simulink model "color_palette_v3"  (Simulink 7.6)
settings: Solver=FixedStepDiscrete  StartTime=0.0  StopTime=0  FixedStep=1/30  RelTol=1e-3
values from neighbouring files (symbols this model uses):
  Iter_Segment_Thresh = 60    [VisionConstants.m]
  Scale_Forward_B = 1    [VisionConstants.m]
  Scale_Forward_G = 1    [VisionConstants.m]
  Scale_Forward_H = .8    (= 0.8)    [VisionConstants.m]
  Scale_Forward_R = 1    [VisionConstants.m]
  Scale_Forward_S = 1    [VisionConstants.m]
  Scale_Forward_V = 2    [VisionConstants.m]
undefined symbols (not defined in the file or in its folder): a_range, b_range, jet, Rec, SDTV
libraries: vipconversions x5, vipgeotforms x3, vipsnks x2, vipsrcs x1
settings Model: Creator=auvt  LastModifiedBy=auvt
settings RTWCC: TargetLang=C++

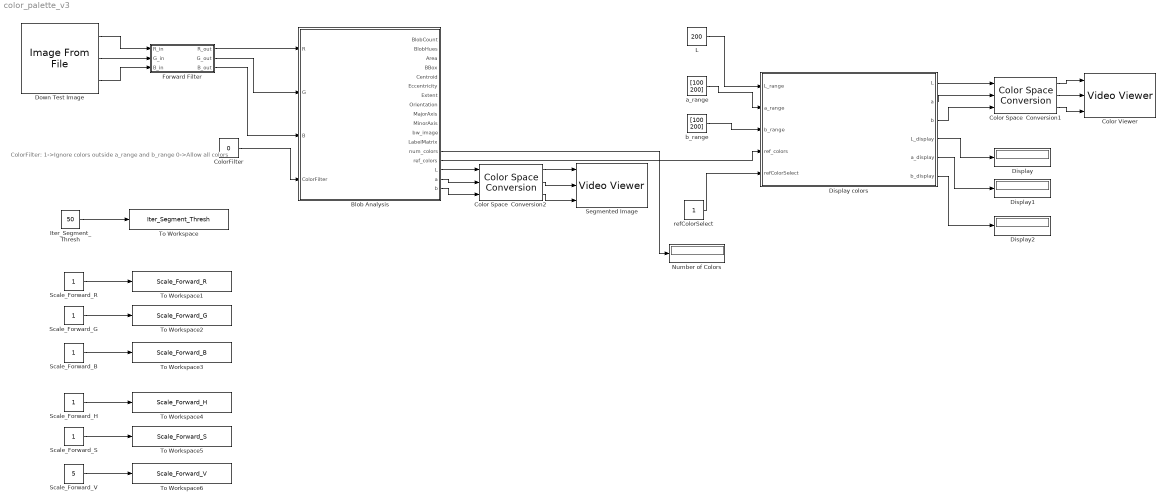
== system color_palette_v3 ==
  note: ColorFilter:
      | 1->Ignore colors outside a_range and b_range
      | 0->Allow all colors
  Blob Analysis : Subsystem
  Color Space  Conversion1 : vipconversions/Color Space  Conversion  conversion=Obsolete  conversionActive=L*a*b* to sR'G'B'  wp_str=D50  rec=Rec. 601 (SDTV)  sys=1125/60/2:1  imagePorts=Separate color signals
  Color Space  Conversion2 : vipconversions/Color Space  Conversion  conversion=Obsolete  conversionActive=L*a*b* to sR'G'B'  wp_str=D50  rec=Rec. 601 (SDTV)  sys=1125/60/2:1  imagePorts=Separate color signals
  Color Viewer : vipsnks/Video Viewer  DialogControllerArgs=DataTag4  inputType=Obsolete7b  imagePorts=Separate color signals  useColorMap=off  colormapValue=jet(256)  specRange=off  minInputVal=0  maxInputVal=255  FigPos=[1526 467 410 300]  AxisZoom=on  trueSizedOnce=off  OpenAtMdlStart=on
  ColorFilter : Constant  Value=0  SampleTime=-1
  Display : Display
  Display colors : Stateflow chart  TreatAsAtomicUnit=on  SystemSampleTime=[1/30 0]
  Display1 : Display
  Display2 : Display
  Down Test Image : vipsrcs/Image From File  Tag=vipblks_nd  DialogController=vipDDGCreate  DialogControllerArgs=DataTag5  SystemSampleTime=-1  FileName=/home/auvt/auvc/src/vision/Test_Images/gate10.bmp  imagePorts=Separate color signals  Ts=-1  ImageDataType=double  Signed=on  WordLength=16  sdImageDataType=uint(8)  FractionLengthMode=User-defined  FractionLength=15  OutPortLabels=R|G|B
  Forward Filter : Subsystem
  Iter_Segment_Thresh : Constant  Value=50  SampleTime=-1
  L : Constant  Value=200  SampleTime=-1
  Number of Colors : Display
  Scale_Forward_B : Constant  SampleTime=-1
  Scale_Forward_G : Constant  SampleTime=-1
  Scale_Forward_H : Constant  SampleTime=-1
  Scale_Forward_R : Constant  SampleTime=-1
  Scale_Forward_S : Constant  SampleTime=-1
  Scale_Forward_V : Constant  Value=5  SampleTime=-1
  Segmented Image : vipsnks/Video Viewer  DialogControllerArgs=DataTag7  inputType=Obsolete7b  imagePorts=Separate color signals  useColorMap=off  colormapValue=jet(256)  specRange=off  minInputVal=0  maxInputVal=255  FigPos=[1521 919 410 300]  AxisZoom=on  trueSizedOnce=off  OpenAtMdlStart=on
  To Workspace : ToWorkspace  VariableName=Iter_Segment_Thresh  SampleTime=-1  SaveFormat=Array
  To Workspace1 : ToWorkspace  VariableName=Scale_Forward_R  SampleTime=-1  SaveFormat=Array
  To Workspace2 : ToWorkspace  VariableName=Scale_Forward_G  SampleTime=-1  SaveFormat=Array
  To Workspace3 : ToWorkspace  VariableName=Scale_Forward_B  SampleTime=-1  SaveFormat=Array
  To Workspace4 : ToWorkspace  VariableName=Scale_Forward_H  SampleTime=-1  SaveFormat=Array
  To Workspace5 : ToWorkspace  VariableName=Scale_Forward_S  SampleTime=-1  SaveFormat=Array
  To Workspace6 : ToWorkspace  VariableName=Scale_Forward_V  SampleTime=-1  SaveFormat=Array
  a_range : Constant  Value=[100 200]  SampleTime=-1
  b_range : Constant  Value=[100 200]  SampleTime=-1
  refColorSelect : Constant  SampleTime=-1
  wires:
  Display colors/1(L) -> Color Space  Conversion1/1
  Display colors/2(a) -> Color Space  Conversion1/2
  Display colors/3(b) -> Color Space  Conversion1/3
  refColorSelect/1 -> Display colors/5(refColorSelect)
  ColorFilter/1 -> Blob Analysis/4(ColorFilter)
  Blob Analysis/14(ref_colors) -> Display colors/4(ref_colors)
  L/1 -> Display colors/1(L_range)
  a_range/1 -> Display colors/2(a_range)
  b_range/1 -> Display colors/3(b_range)
  Display colors/4(L_display) -> Display/1
  Display colors/5(a_display) -> Display1/1
  Display colors/6(b_display) -> Display2/1
  Blob Analysis/13(num_colors) -> Number of Colors/1
  Blob Analysis/15(L) -> Color Space  Conversion2/1
  Blob Analysis/16(a) -> Color Space  Conversion2/2
  Blob Analysis/17(b) -> Color Space  Conversion2/3
  Color Space  Conversion2/1 -> Segmented Image/1
  Color Space  Conversion2/2 -> Segmented Image/2
  Color Space  Conversion2/3 -> Segmented Image/3
  Iter_Segment_Thresh/1 -> To Workspace/1
  Forward Filter/1(R_out) -> Blob Analysis/1(R)
  Forward Filter/2(G_out) -> Blob Analysis/2(G)
  Forward Filter/3(B_out) -> Blob Analysis/3(B)
  Down Test Image/1 -> Forward Filter/1(R_in)
  Down Test Image/2 -> Forward Filter/2(G_in)
  Down Test Image/3 -> Forward Filter/3(B_in)
  Scale_Forward_R/1 -> To Workspace1/1
  Scale_Forward_G/1 -> To Workspace2/1
  Scale_Forward_B/1 -> To Workspace3/1
  Scale_Forward_H/1 -> To Workspace4/1
  Scale_Forward_S/1 -> To Workspace5/1
  Scale_Forward_V/1 -> To Workspace6/1
  Color Space  Conversion1/1 -> Color Viewer/1
  Color Space  Conversion1/2 -> Color Viewer/2
  Color Space  Conversion1/3 -> Color Viewer/3

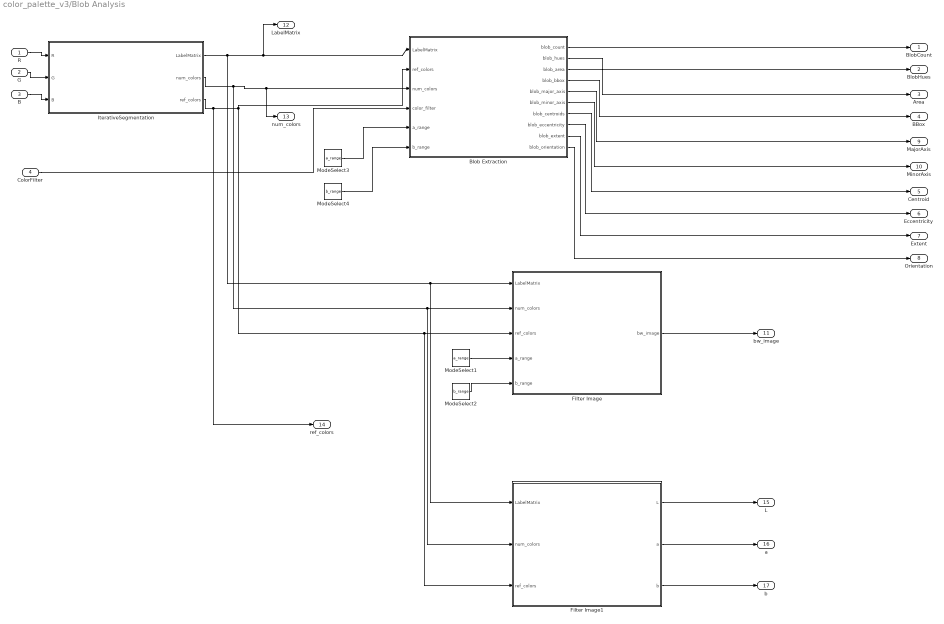
== system color_palette_v3/Blob Analysis ==
  R : Inport
  G : Inport  Port=2
  B : Inport  Port=3
  ColorFilter : Inport  Port=4
  Blob Extraction : Stateflow chart  TreatAsAtomicUnit=on
  Filter Image : Stateflow chart  TreatAsAtomicUnit=on
  Filter Image1 : Stateflow chart  TreatAsAtomicUnit=on
  IterativeSegmentation : Subsystem
      settings: UndoDeleteFcn=Stateflow.SLINSF.SimulinkMan.restorePreDeleteFcn  PreDeleteFcn=Stateflow.SLINSF.SimulinkMan.removePreDeleteFcn
  ModeSelect1 : Constant  Value=a_range  SampleTime=-1
  ModeSelect2 : Constant  Value=b_range  SampleTime=-1
  ModeSelect3 : Constant  Value=a_range  SampleTime=-1
  ModeSelect4 : Constant  Value=b_range  SampleTime=-1
  BlobCount : Outport
  BlobHues : Outport  Port=2
  Area : Outport  Port=3
  BBox : Outport  Port=4
  Centroid : Outport  Port=5
  Eccentricity : Outport  Port=6
  Extent : Outport  Port=7
  Orientation : Outport  Port=8
  MajorAxis : Outport  Port=9
  MinorAxis : Outport  Port=10
  bw_image : Outport  Port=11
  LabelMatrix : Outport  Port=12
  num_colors : Outport  Port=13
  ref_colors : Outport  Port=14
  L : Outport  Port=15
  a : Outport  Port=16
  b : Outport  Port=17
  wires:
  R/1 -> IterativeSegmentation/1(R)
  G/1 -> IterativeSegmentation/2(G)
  B/1 -> IterativeSegmentation/3(B)
  IterativeSegmentation/1(LabelMatrix) -> Blob Extraction/1(LabelMatrix), LabelMatrix/1, Filter Image/1(LabelMatrix), Filter Image1/1(LabelMatrix)
  IterativeSegmentation/2(num_colors) -> Blob Extraction/3(num_colors), num_colors/1, Filter Image/2(num_colors), Filter Image1/2(num_colors)
  IterativeSegmentation/3(ref_colors) -> Blob Extraction/2(ref_colors), Filter Image/3(ref_colors), Filter Image1/3(ref_colors), ref_colors/1
  Blob Extraction/1(blob_count) -> BlobCount/1
  Blob Extraction/2(blob_hues) -> BlobHues/1
  Blob Extraction/3(blob_area) -> Area/1
  Blob Extraction/4(blob_bbox) -> BBox/1
  Blob Extraction/7(blob_centroids) -> Centroid/1
  Blob Extraction/8(blob_eccentricity) -> Eccentricity/1
  Blob Extraction/9(blob_extent) -> Extent/1
  Blob Extraction/10(blob_orientation) -> Orientation/1
  Blob Extraction/5(blob_major_axis) -> MajorAxis/1
  Blob Extraction/6(blob_minor_axis) -> MinorAxis/1
  ModeSelect1/1 -> Filter Image/4(a_range)
  ModeSelect2/1 -> Filter Image/5(b_range)
  Filter Image/1(bw_image) -> bw_image/1
  ModeSelect3/1 -> Blob Extraction/5(a_range)
  ModeSelect4/1 -> Blob Extraction/6(b_range)
  ColorFilter/1 -> Blob Extraction/4(color_filter)
  Filter Image1/1(L) -> L/1
  Filter Image1/2(a) -> a/1
  Filter Image1/3(b) -> b/1

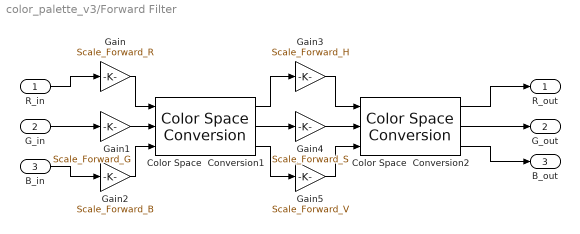
== system color_palette_v3/Forward Filter ==
  R_in : Inport  PortDimensions=Forward_Camera_Dimensions
  G_in : Inport  Port=2  PortDimensions=Forward_Camera_Dimensions
  B_in : Inport  Port=3  PortDimensions=Forward_Camera_Dimensions
  Color Space  Conversion1 : vipconversions/Color Space  Conversion  conversion=Obsolete  conversionActive=R'G'B' to HSV  wp_str=D50  rec=Rec. 601 (SDTV)  sys=1125/60/2:1  imagePorts=Separate color signals
  Color Space  Conversion2 : vipconversions/Color Space  Conversion  conversion=Obsolete  conversionActive=HSV to R'G'B'  wp_str=D50  rec=Rec. 601 (SDTV)  sys=1125/60/2:1  imagePorts=Separate color signals
  Gain : Gain  Gain=Scale_Forward_R
  Gain1 : Gain  Gain=Scale_Forward_G
  Gain2 : Gain  Gain=Scale_Forward_B
  Gain3 : Gain  Gain=Scale_Forward_H
  Gain4 : Gain  Gain=Scale_Forward_S
  Gain5 : Gain  Gain=Scale_Forward_V
  R_out : Outport  OutDataTypeStr=double
  G_out : Outport  Port=2  OutDataTypeStr=double
  B_out : Outport  Port=3  OutDataTypeStr=double
  wires:
  R_in/1 -> Gain/1
  G_in/1 -> Gain1/1
  B_in/1 -> Gain2/1
  Gain/1 -> Color Space  Conversion1/1
  Gain1/1 -> Color Space  Conversion1/2
  Gain2/1 -> Color Space  Conversion1/3
  Color Space  Conversion1/1 -> Gain3/1
  Color Space  Conversion1/2 -> Gain4/1
  Color Space  Conversion1/3 -> Gain5/1
  Gain3/1 -> Color Space  Conversion2/1
  Gain4/1 -> Color Space  Conversion2/2
  Gain5/1 -> Color Space  Conversion2/3
  Color Space  Conversion2/1 -> R_out/1
  Color Space  Conversion2/2 -> G_out/1
  Color Space  Conversion2/3 -> B_out/1

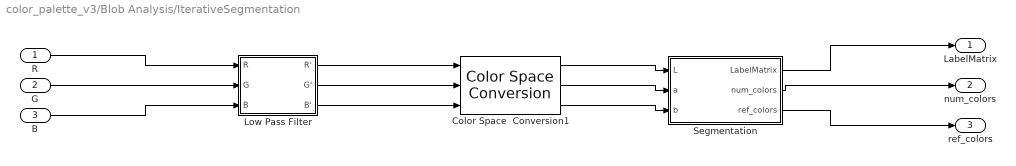
== system color_palette_v3/Blob Analysis/IterativeSegmentation ==
  R : Inport
  G : Inport  Port=2
  B : Inport  Port=3
  Color Space  Conversion1 : vipconversions/Color Space  Conversion  conversion=Obsolete  conversionActive=sR'G'B' to L*a*b*  wp_str=D50  rec=Rec. 601 (SDTV)  sys=1125/60/2:1  imagePorts=Separate color signals
  Low Pass Filter : Subsystem
  Segmentation : Subsystem
  LabelMatrix : Outport
  num_colors : Outport  Port=2
  ref_colors : Outport  Port=3
  wires:
  Segmentation/3(ref_colors) -> ref_colors/1
  Segmentation/2(num_colors) -> num_colors/1
  Segmentation/1(LabelMatrix) -> LabelMatrix/1
  Low Pass Filter/3(B') -> Color Space  Conversion1/3
  Low Pass Filter/2(G') -> Color Space  Conversion1/2
  Low Pass Filter/1(R') -> Color Space  Conversion1/1
  Color Space  Conversion1/3 -> Segmentation/3(b)
  Color Space  Conversion1/2 -> Segmentation/2(a)
  Color Space  Conversion1/1 -> Segmentation/1(L)
  R/1 -> Low Pass Filter/1(R)
  G/1 -> Low Pass Filter/2(G)
  B/1 -> Low Pass Filter/3(B)

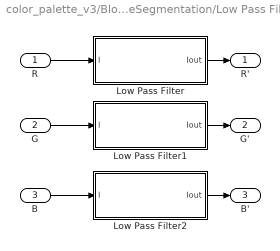
== system color_palette_v3/Blob Analysis/IterativeSegmentation/Low Pass Filter ==
  R : Inport
  G : Inport  Port=2
  B : Inport  Port=3
  Low Pass Filter : Stateflow chart  TreatAsAtomicUnit=on
  Low Pass Filter1 : Stateflow chart  TreatAsAtomicUnit=on
  Low Pass Filter2 : Stateflow chart  TreatAsAtomicUnit=on
  R' : Outport
  G' : Outport  Port=2
  B' : Outport  Port=3
  wires:
  Low Pass Filter/1(Iout) -> R'/1
  Low Pass Filter2/1(Iout) -> B'/1
  Low Pass Filter1/1(Iout) -> G'/1
  B/1 -> Low Pass Filter2/1(I)
  G/1 -> Low Pass Filter1/1(I)
  R/1 -> Low Pass Filter/1(I)

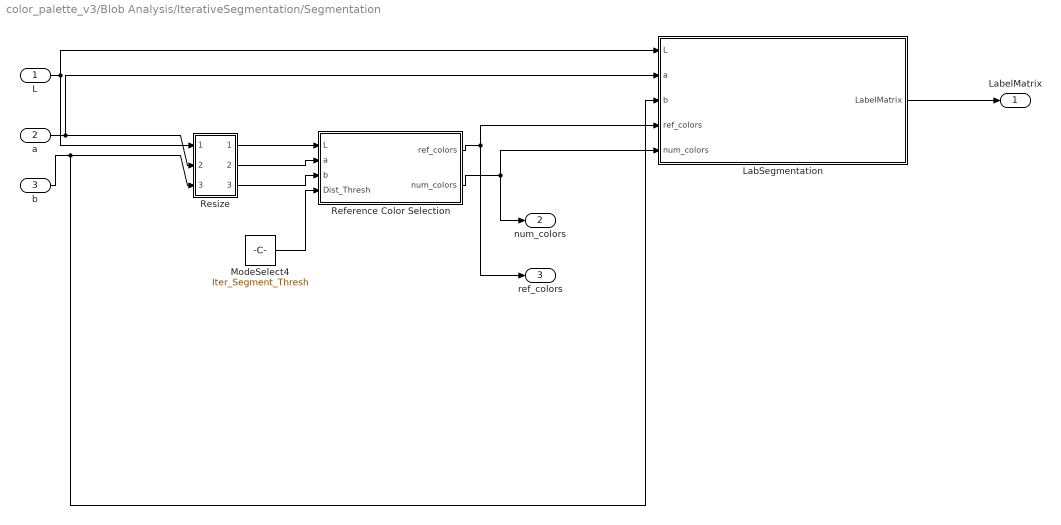
== system color_palette_v3/Blob Analysis/IterativeSegmentation/Segmentation ==
  L : Inport
  a : Inport  Port=2
  b : Inport  Port=3
  LabSegmentation : Stateflow chart  TreatAsAtomicUnit=on
  ModeSelect4 : Constant  Value=Iter_Segment_Thresh  SampleTime=-1
  Reference Color Selection : Stateflow chart  TreatAsAtomicUnit=on
  Resize : Subsystem
  LabelMatrix : Outport
  num_colors : Outport  Port=2
  ref_colors : Outport  Port=3
  wires:
  LabSegmentation/1(LabelMatrix) -> LabelMatrix/1
  Reference Color Selection/2(num_colors) -> LabSegmentation/5(num_colors), num_colors/1
  Reference Color Selection/1(ref_colors) -> ref_colors/1, LabSegmentation/4(ref_colors)
  Resize/3(Out3) -> Reference Color Selection/3(b)
  Resize/2(Out2) -> Reference Color Selection/2(a)
  Resize/1(Out1) -> Reference Color Selection/1(L)
  b/1 -> LabSegmentation/3(b), Resize/3(In3)
  a/1 -> LabSegmentation/2(a), Resize/2(In2)
  L/1 -> LabSegmentation/1(L), Resize/1(In1)
  ModeSelect4/1 -> Reference Color Selection/4(Dist_Thresh)

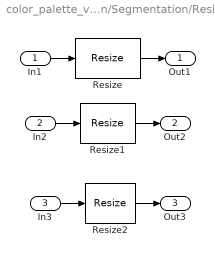
== system color_palette_v3/Blob Analysis/IterativeSegmentation/Segmentation/Resize ==
  In1 : Inport
  In2 : Inport  Port=2
  In3 : Inport  Port=3
  Resize : vipgeotforms/Resize  DialogController=vipDDGCreate  DialogControllerArgs=DataTag0  specify=Number of output rows and columns  rfactor=[]  outCols=25  outRows=25  outRowsCols=[60 80]  interp_method=Bilinear  antialias=on  useROI=off  roiFlag=off  prodOutputMode=Binary point scaling  prodOutputWordLength=32  prodOutputFracLength=10  roundingMode=Nearest  overflowMode=on
  Resize1 : vipgeotforms/Resize  DialogController=vipDDGCreate  DialogControllerArgs=DataTag1  specify=Number of output rows and columns  rfactor=[200 150]  outCols=25  outRows=25  outRowsCols=[60 80]  interp_method=Bilinear  antialias=on  useROI=off  roiFlag=off  prodOutputMode=Binary point scaling  prodOutputWordLength=32  prodOutputFracLength=10  roundingMode=Nearest  overflowMode=on
  Resize2 : vipgeotforms/Resize  DialogController=vipDDGCreate  DialogControllerArgs=DataTag2  specify=Number of output rows and columns  rfactor=[200 150]  outCols=25  outRows=25  outRowsCols=[60 80]  interp_method=Bilinear  antialias=on  useROI=off  roiFlag=off  prodOutputMode=Binary point scaling  prodOutputWordLength=32  prodOutputFracLength=10  roundingMode=Nearest  overflowMode=on
  Out1 : Outport
  Out2 : Outport  Port=2
  Out3 : Outport  Port=3
  wires:
  Resize2/1 -> Out3/1
  In3/1 -> Resize2/1
  Resize1/1 -> Out2/1
  In2/1 -> Resize1/1
  Resize/1 -> Out1/1
  In1/1 -> Resize/1

== matlab function Blob Analysis/Filter Image1 ==
  data: LabelMatrix input double; num_colors input double; ref_colors input double; L output double; a output double; b output double
function [L, a, b] = Display_Image(LabelMatrix, num_colors, ref_colors)


% Initialize
[rows,cols] = size(LabelMatrix);
L = zeros(rows,cols);
a = zeros(rows,cols);
b = zeros(rows,cols);


% Allow only colors in specified range
for r = 1:rows
    for c = 1:cols
        
        L(r,c) = ref_colors(LabelMatrix(r,c), 1);
        a(r,c) = ref_colors(LabelMatrix(r,c), 2);
        b(r,c) = ref_colors(LabelMatrix(r,c), 3);
        
    end
end


return

== matlab function Display colors ==
  data: L_range input double; a_range input double; b_range input double; L output double; a output double; b output double; ref_colors input double; refColorSelect input double; L_display output double; a_display output double; b_display output double
function [L, a, b, L_display, a_display, b_display] = makePalette(L_range, a_range, b_range, ref_colors, refColorSelect)


% Initialize
rows = 200;
cols = 200;

L = zeros(rows, cols);
a = zeros(rows, cols);
b = zeros(rows, cols);


% Display the valid color range gradient
for r = 1:rows
    for c = 1:cols
        
        L(r,c) = L_range(1);
        a(r,c) = a_range(1) + (a_range(2) - a_range(1) )*( (r-1)/(rows-1) );
        b(r,c) = b_range(1) + (b_range(2) - b_range(1) )*( (c-1)/(cols-1) );
        
    end
end


% Place a box in the center of the viewing area with the refColorSelect'th
%   color in ref_colors
for r = 90:110
    for c = 90:110
        L(r,c) = ref_colors(refColorSelect, 1);
        a(r,c) = ref_colors(refColorSelect, 2);
        b(r,c) = ref_colors(refColorSelect, 3);
    end
end


% Display the L, a, b components of the selected color
L_display = ref_colors(refColorSelect, 1);
a_display = ref_colors(refColorSelect, 2);
b_display = ref_colors(refColorSelect, 3);

return

== matlab function Blob Analysis/Blob Extraction ==
  data: LabelMatrix input double; ref_colors input double; num_colors input double; color_filter input double; blob_count output double; blob_hues output double; blob_area output double; blob_bbox output double; blob_major_axis output double; blob_minor_axis output double; blob_centroids output double; blob_eccentricity output double; blob_extent output double; blob_orientation output double; a_range input double; b_range input double
function [blob_count, blob_hues, blob_area, blob_bbox, blob_major_axis, blob_minor_axis, blob_centroids, blob_eccentricity, blob_extent, blob_orientation] = GetBlobInfo(LabelMatrix, ref_colors, num_colors, color_filter, a_range, b_range)

% This function extracts 
% Input
%   

% Initialize
max_num_blobs = 50;
min_blob_area = 5;

[rows, cols] = size(LabelMatrix);
LogicMatrix = false(rows,cols);

blob_count = 0;
blob_hues = zeros(3,max_num_blobs);

blob_area = -1.*ones(1,max_num_blobs);
blob_bbox = zeros(4,max_num_blobs);
blob_major_axis = zeros(1,max_num_blobs);
blob_minor_axis = zeros(1,max_num_blobs);
blob_centroids = zeros(2,max_num_blobs);
blob_eccentricity = zeros(1,max_num_blobs);
blob_extent = zeros(1,max_num_blobs);
blob_orientation = zeros(1,max_num_blobs);


% Input hblob, a matrix containing [Area, blob_centroids, Eccentricity] for each
% identified blob
persistent hblob
if isempty(hblob)
    hblob = video.BlobAnalysis('AreaOutputPort',true,'CentroidOutputPort',true,...
        'BoundingBoxOutputPort',true,'MajorAxisLengthOutputPort',true,'MinorAxisLengthOutputPort',true,...
        'OrientationOutputPort',true,...
        'EccentricityOutputPort',true,'ExtentOutputPort',true,'NumBlobsOutputPort',true,...
        'MinimumBlobAreaSource','Property','MinimumBlobArea', min_blob_area);
end


% Calculate geometric information about the blobs
%
% LogicMatrix is a binary version of LabelMatrix, with ones at all
%   locations for which color values are k, and zeros everywhere else
for k = 1:num_colors

    a = ref_colors(k, 2);
    b = ref_colors(k, 3);

    if( color_filter == 1 && a >= a_range(1,5) && a <= a_range(2,5) && b >= b_range(1,5) && b <= b_range(2,5) )

        for i = 1:rows
            for j = 1:cols
                if(LabelMatrix(i,j) ~= k)
                    LogicMatrix(i,j) = false;
                else
                    LogicMatrix(i,j) = true;
                end
            end
        end

        [TArea,TCentroid,TBBox,TMajorAxis,TMinorAxis,TOrientation,TEccent,TExtent,TNumBlobs] = step(hblob,LogicMatrix);

        for i = 1:TNumBlobs
            if(blob_count + TNumBlobs <= max_num_blobs)

                blob_centroids(1,blob_count+i) = TCentroid(1,i);
                blob_centroids(2,blob_count+i) = TCentroid(2,i);

                ii = round(blob_centroids(1,blob_count+i));
                jj = round(blob_centroids(2,blob_count+i));

                blob_hues(1,blob_count+i) = ref_colors( LabelMatrix(ii,jj), 1 );
                blob_hues(2,blob_count+i) = ref_colors( LabelMatrix(ii,jj), 2 );
                blob_hues(3,blob_count+i) = ref_colors( LabelMatrix(ii,jj), 3 );

                blob_area(blob_count+i) = TArea(i);
                blob_bbox(blob_count+i) = TBBox(i);
                blob_major_axis(blob_count+i) = TMajorAxis(i);
                blob_minor_axis(blob_count+i) = TMinorAxis(i);
                blob_eccentricity(blob_count+i) = TEccent(i);
                blob_extent(blob_count+i) = TExtent(i);
                blob_orientation(blob_count+i) = TOrientation(i);

            end
        end

        blob_count = blob_count + double(TNumBlobs);

    end
    
end


return

== matlab function Blob Analysis/Filter Image ==
  data: LabelMatrix input double; num_colors input double; ref_colors input double; bw_image output double; a_range input double; b_range input double
function bw_image = Filter_Image(LabelMatrix, num_colors, ref_colors, a_range, b_range)


% Initialize
[rows,cols] = size(LabelMatrix);
bw_image = zeros(rows,cols);


% Allow only colors in specified range
for r = 1:rows
    for c = 1:cols
        
        a = ref_colors(LabelMatrix(r,c), 2);
        b = ref_colors(LabelMatrix(r,c), 3);
        
        if( a >= a_range(1,5) && a <= a_range(2,5) && b >= b_range(1,5) && b <= b_range(2,5) )
            bw_image(r,c) = 1;
        end
        
    end
end


return

== matlab function Blob Analysis/IterativeSegmentation/Low Pass Filter/Low Pass Filter ==
  data: I input double; Iout output double
function Iout = GaussianBlurr(I)
% This function calculates the gaussian blur of an intensity image

sigma = sqrt(2);

Grows = 3;    % Gaussian matrix rows
Gcols = 3;    % Gaussian matrix columns

[Irows Icols] = size(I);

Iout = double(zeros(Irows,Icols));

Trows = Irows - Grows + 1;
Tcols = Icols - Gcols + 1;
Itemp = double(zeros(Trows,Tcols));

G = zeros(Grows,Gcols);

FirstRow = ceil(-Grows/2);
LastRow = floor(Grows/2);
FirstCol = ceil(-Gcols/2);
LastCol = floor(Gcols/2);
Gsum = 0;
for i=FirstRow:LastRow
    for j = FirstCol:LastCol
        G(i-FirstRow+1,j-FirstCol+1) = exp(-(j*j+i*i)/(2*sigma*sigma));
        Gsum = Gsum + G(i-FirstRow+1,j-FirstCol+1);
    end
end

G = G./Gsum;

Itemp = conv2(double(I),double(G),'valid');

% reflect boundaries to keep image the same size
% top
Iout((1:LastRow),(LastCol+1:Icols-LastCol)) = Itemp((1:LastRow),(1:Tcols));
% bottom
Iout((Irows-LastRow+1:Irows),(LastCol+1:Icols-LastCol)) = Itemp((Trows-LastRow+1:Trows),(1:Tcols));
% left
Iout((1+LastRow:Irows-LastRow),(1:LastCol)) = Itemp((1:Trows),(1:LastCol));
% right
Iout((1+LastRow:Irows-LastRow),(Icols-LastCol+1:Icols)) = Itemp((1:Trows),(Tcols-LastCol+1:Tcols));
% center
Iout((1+LastRow:Irows-LastRow),(1+LastCol:Icols-LastCol)) = Itemp;
% top left corner
Iout(1:LastRow,1:LastCol) = Itemp(1:LastRow,1:LastCol);
% top right corner
Iout(1:LastRow,Icols-LastCol:Icols) = Itemp(1:LastRow,Tcols-LastCol:Tcols);
% bottom left corner
Iout(Irows-LastRow:Irows,1:LastCol) = Itemp(Trows-LastRow:Trows,1:LastCol);
% bottom right corner
Iout(Irows-LastRow:Irows,Icols-LastCol:Icols) = Itemp(Trows-LastRow:Trows,Tcols-LastCol:Tcols);

return

== matlab function Blob Analysis/IterativeSegmentation/Low Pass Filter/Low Pass Filter1 ==
  data: I input double; Iout output double
function Iout = GaussianBlurr(I)
% This function calculates the gaussian blur of an intensity image

sigma = sqrt(2);

Grows = 3;    % Gaussian matrix rows
Gcols = 3;    % Gaussian matrix columns

[Irows Icols] = size(I);

Iout = double(zeros(Irows,Icols));

Trows = Irows - Grows + 1;
Tcols = Icols - Gcols + 1;
Itemp = double(zeros(Trows,Tcols));

G = zeros(Grows,Gcols);

FirstRow = ceil(-Grows/2);
LastRow = floor(Grows/2);
FirstCol = ceil(-Gcols/2);
LastCol = floor(Gcols/2);
Gsum = 0;
for i=FirstRow:LastRow
    for j = FirstCol:LastCol
        G(i-FirstRow+1,j-FirstCol+1) = exp(-(j*j+i*i)/(2*sigma*sigma));
        Gsum = Gsum + G(i-FirstRow+1,j-FirstCol+1);
    end
end

G = G./Gsum;

Itemp = conv2(double(I),double(G),'valid');

% reflect boundaries to keep image the same size
% top
Iout((1:LastRow),(LastCol+1:Icols-LastCol)) = Itemp((1:LastRow),(1:Tcols));
% bottom
Iout((Irows-LastRow+1:Irows),(LastCol+1:Icols-LastCol)) = Itemp((Trows-LastRow+1:Trows),(1:Tcols));
% left
Iout((1+LastRow:Irows-LastRow),(1:LastCol)) = Itemp((1:Trows),(1:LastCol));
% right
Iout((1+LastRow:Irows-LastRow),(Icols-LastCol+1:Icols)) = Itemp((1:Trows),(Tcols-LastCol+1:Tcols));
% center
Iout((1+LastRow:Irows-LastRow),(1+LastCol:Icols-LastCol)) = Itemp;
% top left corner
Iout(1:LastRow,1:LastCol) = Itemp(1:LastRow,1:LastCol);
% top right corner
Iout(1:LastRow,Icols-LastCol:Icols) = Itemp(1:LastRow,Tcols-LastCol:Tcols);
% bottom left corner
Iout(Irows-LastRow:Irows,1:LastCol) = Itemp(Trows-LastRow:Trows,1:LastCol);
% bottom right corner
Iout(Irows-LastRow:Irows,Icols-LastCol:Icols) = Itemp(Trows-LastRow:Trows,Tcols-LastCol:Tcols);

return

== matlab function Blob Analysis/IterativeSegmentation/Low Pass Filter/Low Pass Filter2 ==
  data: I input double; Iout output double
function Iout = GaussianBlurr(I)
% This function calculates the gaussian blur of an intensity image

sigma = sqrt(2);

Grows = 3;    % Gaussian matrix rows
Gcols = 3;    % Gaussian matrix columns

[Irows Icols] = size(I);

Iout = double(zeros(Irows,Icols));

Trows = Irows - Grows + 1;
Tcols = Icols - Gcols + 1;
Itemp = double(zeros(Trows,Tcols));

G = zeros(Grows,Gcols);

FirstRow = ceil(-Grows/2);
LastRow = floor(Grows/2);
FirstCol = ceil(-Gcols/2);
LastCol = floor(Gcols/2);
Gsum = 0;
for i=FirstRow:LastRow
    for j = FirstCol:LastCol
        G(i-FirstRow+1,j-FirstCol+1) = exp(-(j*j+i*i)/(2*sigma*sigma));
        Gsum = Gsum + G(i-FirstRow+1,j-FirstCol+1);
    end
end

G = G./Gsum;

Itemp = conv2(double(I),double(G),'valid');

% reflect boundaries to keep image the same size
% top
Iout((1:LastRow),(LastCol+1:Icols-LastCol)) = Itemp((1:LastRow),(1:Tcols));
% bottom
Iout((Irows-LastRow+1:Irows),(LastCol+1:Icols-LastCol)) = Itemp((Trows-LastRow+1:Trows),(1:Tcols));
% left
Iout((1+LastRow:Irows-LastRow),(1:LastCol)) = Itemp((1:Trows),(1:LastCol));
% right
Iout((1+LastRow:Irows-LastRow),(Icols-LastCol+1:Icols)) = Itemp((1:Trows),(Tcols-LastCol+1:Tcols));
% center
Iout((1+LastRow:Irows-LastRow),(1+LastCol:Icols-LastCol)) = Itemp;
% top left corner
Iout(1:LastRow,1:LastCol) = Itemp(1:LastRow,1:LastCol);
% top right corner
Iout(1:LastRow,Icols-LastCol:Icols) = Itemp(1:LastRow,Tcols-LastCol:Tcols);
% bottom left corner
Iout(Irows-LastRow:Irows,1:LastCol) = Itemp(Trows-LastRow:Trows,1:LastCol);
% bottom right corner
Iout(Irows-LastRow:Irows,Icols-LastCol:Icols) = Itemp(Trows-LastRow:Trows,Tcols-LastCol:Tcols);

return

== matlab function Blob Analysis/IterativeSegmentation/Segmentation/LabSegmentation ==
  data: L input double; LabelMatrix output double; a input double; b input double; ref_colors input double; num_colors input double
function LabelMatrix  = LabSegmentation(L,a,b,ref_colors,num_colors)
% This function generates the label matrix

[rows cols] = size(L);

Lout = zeros(rows,cols);
aout = zeros(rows,cols);
bout = zeros(rows,cols);

LabelMatrix = zeros(rows,cols);

for i = 1:rows
    for j = 1:cols
        min_dist = 1000;
        index = 1;
        for k = 1:num_colors
            dist = sqrt((ref_colors(k,1) - L(i,j))^2 + (ref_colors(k,2) - a(i,j))^2 + (ref_colors(k,3) - b(i,j))^2);
            if(dist < min_dist)
                min_dist = double(dist);
                index = k;
            end
        end
        LabelMatrix(i,j) = index;
    end
end

for i = 1:rows
    for j = 1:cols
        Lout(i,j) = ref_colors(LabelMatrix(i,j),1);
        aout(i,j) = ref_colors(LabelMatrix(i,j),2);
        bout(i,j) = ref_colors(LabelMatrix(i,j),3);
    end
end

cow = 1;

return

== matlab function Blob Analysis/IterativeSegmentation/Segmentation/Reference Color Selection ==
  data: L input double; ref_colors output double; a input double; b input double; num_colors output double; Dist_Thresh input double
function [ref_colors, num_colors] = Segmentation(L,a,b,Dist_Thresh)
% This function tries segmentation by adding new reference colors everytime
% a pixel is found with a distance greater than a certain amount from
% every other reference color

[rows cols] = size(L);

Dist_Threshold = Dist_Thresh;% L = 0 to 100, a = -100 to 100, b = -100 to 100
                    % max dist = 300 -> 60/300 is 20%
x = 1;  % coefficients determining distance calculation
y = 1.5;
z = 1.5;

max_num_colors = 50;
ref_colors = zeros(max_num_colors,3);   % At most 50 different reference colors
LabelMatrix = zeros(rows,cols);
num_colors = 1;

center_row = floor(rows/2);
center_col = floor(cols/2);

% Define first reference color to be colr
ref_colors(1,:) = [L(center_row,center_col) a(center_row,center_col) b(center_row,center_col)];

flag = 0;
i = 1;
j = 1;
while(i <= rows)        % perform initial segmentation
    while(i <= rows && flag == 0)
        while(j <= cols && flag == 0)
            k = 1;
            min_dist = 1000;
            index = 1;
            while(k <= num_colors)
                dist = sqrt(x*(ref_colors(k,1) - L(i,j))^2 + y*(ref_colors(k,2) - a(i,j))^2 + z*(ref_colors(k,3) - b(i,j))^2);
                if(min_dist > dist)
                    min_dist = double(dist);
                    index = k;
                end
                k = k + 1;
            end
            if(j == 117)
                cow = 1;
            end
            if(min_dist > Dist_Threshold && num_colors < max_num_colors)
                ref_colors(num_colors+1,:) = [L(i,j) a(i,j) b(i,j)];
                num_colors = num_colors + 1;
                flag = 1;
                i = 0;
                j = 0;
            else
                LabelMatrix(i,j) = index;
            end
            j = j + 1;
        end
        j = 1;
        i = i + 1;
    end
    flag = 0;
end

% Go through image once more to get more accurate values for the different regions
ref_color_L_avg = zeros(50,1);
ref_color_a_avg = zeros(50,1);
ref_color_b_avg = zeros(50,1);
color_count = zeros(50,1);
for i = 1:rows
    for j = 1:cols
        index = LabelMatrix(i,j);
        ref_color_L_avg(index) = ref_color_L_avg(index) + L(i,j);
        ref_color_a_avg(index) = ref_color_a_avg(index) + a(i,j);
        ref_color_b_avg(index) = ref_color_b_avg(index) + b(i,j);
        color_count(index) = color_count(index) + 1;
    end
end
ref_color_L_avg = ref_color_L_avg ./ color_count;
ref_color_a_avg = ref_color_a_avg ./ color_count;
ref_color_b_avg = ref_color_b_avg ./ color_count;

for i = 1:num_colors
    ref_colors(i,1) = ref_color_L_avg(i);
    ref_colors(i,2) = ref_color_a_avg(i);
    ref_colors(i,3) = ref_color_b_avg(i);
end

return
